simulink model "PKM_Planar_Testbench_2018"  (R2024a)
settings: Solver=FixedStepDiscrete  StartTime=0.0  StopTime=inf  FixedStep=param.t_sample  RelTol=1e-3
undefined symbols (not defined in the file or in its folder): max_qa, min_qa, param, slave3
libraries: Cust_Library_planarPKM x54, simulink_extras x27, dspswit3 x24, simulink x22, etherlab_lib x12
(part 4 of 6)

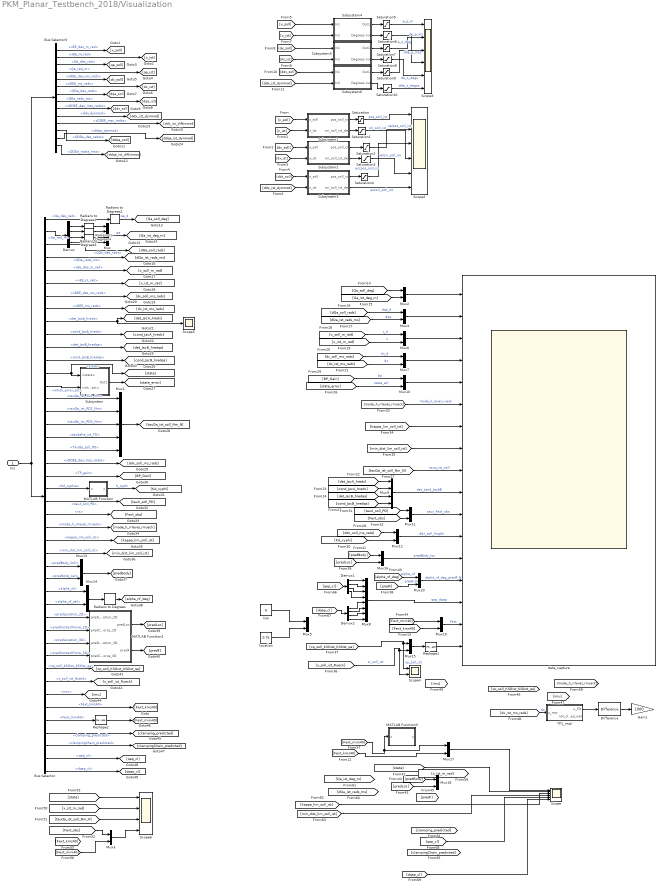
== system PKM_Planar_Testbench_2018/Visualization ==
  In1 : Inport
  Bus Selector : BusSelector  OutputSignals=Logical data.Qa_des_rad,Kinematics_currentValues.Qa_rad_m,Logical data.QDa_des_rads,Differential kinematics - current values.QDa_rads_ms,Logical data.xEE_des_m_rad,Kinematics_currentValues.xEE_m_rad,Logical data.xDEE_des_ms_rads,Differential kinematics - current values.xDEE_ms_rads,Differential kinematics - current values.det_JacA_hredx,Differential kinematics - current values.cond_JacA_hredx,Differential kinematics - current values.det_JacB_hredqa,Differential kinematics - current values.cond_JacB_hredqa,Logical data.state,Logical data.which_error_act,Messdaten.tauQa_ist_RD1_Nm,Messdaten.tauQa_ist_RD2_Nm,Messdaten.tauQa_ist_RD3_Nm,Messdaten.taudelta_ist_TD,PD_Controller.TauQa_soll_PD,Logical data.xDDEE_des_mss_radss,Controlpanel.TP_gain,PD_Controller.Kd_xyphie,PD_Controller.tauX_soll_PD,Beobachter.rx,PD_Controller.mode_h_rrlevel_rrrueck,PD_Controller.kappa_lim_soll_ist,PD_Controller.min_dist_lim_soll_ist,Beobachter.predBody_Coll,Beobachter.predbody_sel,Beobachter.alpha_nf,PD_Controller.alpha_nf_sel,Beobachter.predLocation_2D,Beobachter.predContactForce_2D,Beobachter.predLocation_3D,Beobachter.predContactForce_3D,PD_Controller.xp_soll_KSGist_KS0ist_qa,PD_Controller.x_soll_ist_Rueck,Messdaten.imu,Messdaten.Fext_kms40,Messdaten.Fext_mini40,Beobachter.clamping_predicted,Beobachter.clampingChain_predicted,PD_Controller.qap_cl,PD_Controller.dqap_cl
  Bus Selector3 : BusSelector  OutputSignals=Logical data.xEE_des_m_rad,Kinematics_currentValues.xEE_m_rad,Logical data.Qa_des_rad,Kinematics_currentValues.Qa_rad_m,Logical data.xDEE_des_ms_rads,Differential kinematics - current values.xDEE_ms_rads,Logical data.QDa_des_rads,Differential kinematics - current values.QDa_rads_ms,Logical data.xDDEE_des_mss_radss,Dynamik.ddx_dynmod,Differential kinematics - current values.xDDEE_mss_radss,Logical data.QDDa_des_radss,Dynamik.ddqa_dynmod,Differential kinematics - current values.QDDa_radss_mss
  Demux : Demux
  Demux1 : Demux
  Demux2 : Demux
  Difference : simulink/Discrete/Difference  ICPrevInput=0  OutMin=[]  OutMax=[]  OutDataType=fixdt(1, 16)  OutScaling=2^-10  DoSatur=off
  Gain1 : Gain  Gain=1000
  MATLAB Function : MATLAB Function  TreatAsAtomicUnit=on
  MATLAB Function2 : MATLAB Function  TreatAsAtomicUnit=on
  MATLAB Function3 : MATLAB Function  TreatAsAtomicUnit=on
  Mux : Mux
  Mux1 : Mux  Inputs=5
  Mux{2..7,10..20} (17 alike) : Mux  Inputs=2
  Mux8 : Mux  Inputs=8
  Mux9 : Mux
  Radians to Degrees{,1..4} (5 alike) : simulink_extras/Transformations/Radians to Degrees
  Reshape1 : Reshape
  Reshape2 : Reshape
  Saturation{,5,7,9} (4 alike) : Saturate  UpperLimit=0.35  LowerLimit=-0.35
  Saturation{1,3,6,8,10} (5 alike) : Saturate  UpperLimit=45  LowerLimit=-45
  Saturation2 : Saturate  UpperLimit=2  LowerLimit=-2
  Saturation4 : Saturate  UpperLimit=30  LowerLimit=-30
  Scope : Scope  NumInputPorts=6
  Scope2 : Scope  NumInputPorts=6
  Scope3 : Scope  NumInputPorts=6
  Scope4 : Scope  NumInputPorts=2
  Scope5 : Scope
  Scope6 : Scope  NumInputPorts=4
  Subsystem : Subsystem
  Subsystem1 : Subsystem
  Subsystem2 : Subsystem
  Subsystem3 : Subsystem
  Subsystem4 : Subsystem
  Subsystem5 : Subsystem
  Subsystem6 : Subsystem
  TP1_impl : Subsystem
  data_capture : Scope  NumInputPorts=17
  link : Constant  Value=6  SampleTime=-1
  location : Constant  Value=0.75  SampleTime=-1
  wires:
  Bus Selector/1 -> Radians to Degrees2/1  "<Qa_des_rad>"
  Bus Selector/16 -> Mux1/2  "<tauQa_ist_RD2_Nm>"
  Bus Selector/15 -> Mux1/1  "<tauQa_ist_RD1_Nm>"
  Bus Selector/17 -> Mux1/3  "<tauQa_ist_RD3_Nm>"
  Bus Selector/18 -> Mux1/4  "<taudelta_ist_TD>"
  Bus Selector/13 -> Subsystem/1(<state>), [state]  "<state>"
  Bus Selector/14 -> Subsystem/2(<which_error_act>)  "<which_error_act>"
  Bus Selector/22 -> MATLAB Function/1(u)  "<Kd_xyphie>"
  Bus Selector/24 -> [Fext_obs]  "<rx>"
  Bus Selector3/10 -> [ddx_ist_dynmod]  "<ddx_dynmod>"
  Bus Selector3/13 -> [ddqa_ist_dynmod]  "<ddqa_dynmod>"
  In1/1 -> Bus Selector3/1, Bus Selector/1
  Bus Selector3/1 -> [x_soll]  "<xEE_des_m_rad>"
  Bus Selector3/2 -> [x_ist]  "<xEE_m_rad>"
  Bus Selector3/3 -> [qa_soll]  "<Qa_des_rad>"
  Bus Selector3/4 -> [qa_ist]  "<Qa_rad_m>"
  Bus Selector3/6 -> [dx_ist]  "<xDEE_ms_rads>"
  Bus Selector3/5 -> [dx_soll]  "<xDEE_des_ms_rads>"
  Bus Selector3/7 -> [dqa_soll]  "<QDa_des_rads>"
  Bus Selector3/8 -> [dqa_ist]  "<QDa_rads_ms>"
  Bus Selector3/9 -> [ddx_soll]  "<xDDEE_des_mss_radss>"
  Bus Selector3/11 -> [ddx_ist_difkinmod]  "<xDDEE_mss_radss>"
  Bus Selector3/12 -> [ddqa_soll]  "<QDDa_des_radss>"
  Bus Selector3/14 -> [ddqa_ist_difkinmod]  "<QDDa_radss_mss>"
  [x_soll] -> Subsystem1/1(x_soll)
  [x_ist] -> Subsystem1/2(x_ist)
  [dx_ist] -> Subsystem2/2(x_ist)
  [dx_soll] -> Subsystem2/1(x_soll)
  [ddx_soll] -> Subsystem3/1(x_soll)
  [ddx_ist_dynmod] -> Subsystem3/2(x_ist)
  Subsystem1/1(pos_soll_ist) -> Saturation/1
  Subsystem2/1(pos_soll_ist) -> Saturation2/1
  Subsystem3/1(pos_soll_ist) -> Saturation4/1
  Subsystem1/2(ori_soll_ist_deg) -> Saturation1/1
  Subsystem2/2(ori_soll_ist_deg) -> Saturation3/1
  Subsystem3/2(ori_soll_ist_deg) -> Scope2/6  "accori_soll_ist"
  Saturation/1 -> Scope2/1  "pos_soll_ist"
  Saturation1/1 -> Scope2/4  "ori_soll_ist"
  Saturation2/1 -> Scope2/2  "velpos_soll_ist"
  Saturation3/1 -> Scope2/5  "velori_soll_ist"
  Saturation4/1 -> Scope2/3  "accpos_soll_ist"
  Saturation5/1 -> Scope3/1  "e_p_m"
  [x_soll] -> Subsystem4/1(In1)
  [x_ist] -> Subsystem4/2(In2)
  Subsystem4/1(Out1) -> Saturation5/1
  Subsystem4/2(Degrees out) -> Saturation6/1
  Saturation6/1 -> Scope3/4  "e_o_deg"
  Saturation8/1 -> Scope3/5  "de_o_degs"
  Subsystem5/2(Degrees out) -> Saturation8/1
  Subsystem5/1(Out1) -> Saturation7/1
  [dx_ist] -> Subsystem5/2(In2)
  [dx_soll] -> Subsystem5/1(In1)
  Saturation7/1 -> Scope3/2  "de_p_ms"
  Saturation9/1 -> Scope3/3  "dde_p_mss"
  [ddx_soll] -> Subsystem6/1(In1)
  [ddx_ist_dynmod] -> Subsystem6/2(In2)
  Subsystem6/1(Out1) -> Saturation9/1
  Subsystem6/2(Degrees out) -> Saturation10/1
  Saturation10/1 -> Scope3/6  "dde_o_degss"
  [Fext_mini40] -> MATLAB Function3/1(u), Mux17/1
  Radians to Degrees2/1 -> [Qa_soll_deg]  "qa_d"
  Bus Selector/3 -> [dQa_soll_rads]  "<QDa_des_rads>"
  Bus Selector/2 -> Demux/1  "<Qa_rad_m>"
  Demux/1 -> Radians to Degrees1/1
  Demux/2 -> Radians to Degrees3/1
  Demux/3 -> Radians to Degrees4/1
  Radians to Degrees4/1 -> Mux/3
  Radians to Degrees3/1 -> Mux/2
  Radians to Degrees1/1 -> Mux/1
  Demux/4 -> Mux/4
  Mux/1 -> [Qa_ist_deg_m]  "qa"
  Bus Selector/4 -> [dQa_ist_rads_ms]  "<QDa_rads_ms>"
  Bus Selector/5 -> [x_soll_m_rad]  "<xEE_des_m_rad>"
  Bus Selector/6 -> [x_ist_m_rad]  "<xEE_m_rad>"
  Bus Selector/7 -> [dx_soll_ms_rads]  "<xDEE_des_ms_rads>"
  Bus Selector/8 -> [dx_ist_ms_rads]  "<xDEE_ms_rads>"
  Bus Selector/9 -> Scope5/1, [det_JacA_hredx]  "<det_JacA_hredx>"
  Bus Selector/10 -> [cond_JacA_hredx]  "<cond_JacA_hredx>"
  Bus Selector/11 -> [det_JacB_hredqa]  "<det_JacB_hredqa>"
  Bus Selector/12 -> [cond_JacB_hredqa]  "<cond_JacB_hredqa>"
  Subsystem/1(Out1) -> [state_error]
  Mux1/1 -> [tauQa_ist_soll_Nm_N]
  Bus Selector/19 -> Mux1/5  "<TauQa_soll_PD>"
  Bus Selector/20 -> [ddx_soll_ms_rads]  "<xDDEE_des_mss_radss>"
  Bus Selector/21 -> [BP_Gain]  "<TP_gain>"
  MATLAB Function/1(y) -> [Kd_xyphi]  "K_xyphi"
  Bus Selector/23 -> [tauX_soll_PD]  "<tauX_soll_PD>"
  [Qa_soll_deg] -> Mux2/1
  [Qa_ist_deg_m] -> Mux2/2
  [dQa_soll_rads] -> Mux4/1  "dqa_d"
  [dQa_ist_rads_ms] -> Mux4/2  "dqa"
  [dx_ist_ms_rads] -> Mux7/2  "dx"
  [dx_soll_ms_rads] -> Mux7/1  "dx_d"
  [x_ist_m_rad] -> Mux6/2  "x"
  [x_soll_m_rad] -> Mux6/1  "x_d"
  [det_JacA_hredx] -> Mux9/1
  [cond_JacA_hredx] -> Mux9/2
  [det_JacB_hredqa] -> Mux9/3
  [cond_JacB_hredqa] -> Mux9/4
  Bus Selector/25 -> [mode_h_rrlevel_rrrueck]  "<mode_h_rrlevel_rrrueck>"
  Bus Selector/26 -> [kappa_lim_soll_ist]  "<kappa_lim_soll_ist>"
  Bus Selector/27 -> [min_dist_lim_soll_ist]  "<min_dist_lim_soll_ist>"
  Mux2/1 -> data_capture/1
  Mux4/1 -> data_capture/2
  Mux6/1 -> data_capture/3
  Mux7/1 -> data_capture/4
  [BP_Gain] -> Mux10/1  "bp"
  [state_error] -> Mux10/2  "state_err"
  [tauX_soll_PD] -> Mux11/1
  [Fext_obs] -> Mux11/2
  [ddx_soll_ms_rads] -> Mux12/1
  [Kd_xyphi] -> Mux12/2
  Mux10/1 -> data_capture/5
  [mode_h_rrlevel_rrrueck] -> data_capture/6  "mode_h_level_rueck"
  [kappa_lim_soll_ist] -> data_capture/7
  [min_dist_lim_soll_ist] -> data_capture/8
  [tauQa_ist_soll_Nm_N] -> data_capture/9  "tauq_ist_soll"
  Mux9/1 -> data_capture/10  "det_cond_JacAB"
  Mux11/1 -> data_capture/11  "taux_Fext_obs"
  Mux12/1 -> data_capture/12  "ddx_soll_Kxyphi"
  Bus Selector/28 -> Mux13/1  "<predBody_Coll>"
  Bus Selector/29 -> Mux13/2  "<predbody_sel>"
  Mux13/1 -> [predBody]
  Bus Selector/30 -> Mux14/1  "<alpha_nf>"
  Bus Selector/32 -> MATLAB Function2/1(predLocation_2D)  "<predLocation_2D>"
  Bus Selector/31 -> Mux14/2  "<alpha_nf_sel>"
  Mux14/1 -> Radians to Degrees/1
  Radians to Degrees/1 -> [alpha_nf_deg]
  Bus Selector/33 -> MATLAB Function2/2(predContactForce_2D)  "<predContactForce_2D>"
  Bus Selector/34 -> MATLAB Function2/3(predLocation_3D)  "<predLocation_3D>"
  Bus Selector/35 -> MATLAB Function2/4(predContactForce_3D)  "<predContactForce_3D>"
  MATLAB Function2/1(predLoc) -> [predLoc]
  MATLAB Function2/2(predF) -> [predF]
  Bus Selector/37 -> [x_soll_ist_Rueck]  "<x_soll_ist_Rueck>"
  [predBody] -> Mux16/1
  [predLoc] -> Mux16/2
  Mux16/1 -> data_capture/13  "predBody_loc"
  [Fext_kms40] -> Mux19/2
  Bus Selector/36 -> [xp_soll_KSGist_KS0ist_qa]  "<xp_soll_KSGist_KS0ist_qa>"
  [xp_soll_KSGist_KS0ist_qa] -> Scope4/1, Mux15/1  "xp_soll_ist"
  [x_soll_ist_Rueck] -> Scope4/2, Mux15/2  "xr_soll_ist"
  [state] -> Scope/2
  Mux17/1 -> Scope/1
  [predLoc] -> Mux18/2
  [predBody] -> Mux18/1
  Bus Selector/38 -> [imu]  "<imu>"
  [dx_ist_ms_rads] -> TP1_impl/1(u_raw)  "dx"
  TP1_impl/1(u_filt) -> Difference/1
  Difference/1 -> Gain1/1
  Mux15/1 -> Reshape1/1
  [x_ist_m_rad] -> Scope6/2
  [tauQa_ist_soll_Nm_N] -> Scope6/3
  [Fext_obs] -> Mux3/1
  [state] -> Scope6/1
  Mux19/1 -> data_capture/16  "Fext"
  [Fext_mini40] -> Mux19/1
  Bus Selector/39 -> [Fext_kms40]  "<Fext_kms40>"
  Bus Selector/40 -> Reshape2/1  "<Fext_mini40>"
  [Fext_mini40] -> Mux3/2
  Mux3/1 -> Scope6/4
  link/1 -> Mux5/1
  location/1 -> Mux5/2
  Reshape1/1 -> data_capture/17
  [kappa_lim_soll_ist] -> Scope/3
  [min_dist_lim_soll_ist] -> Scope/4
  Bus Selector/41 -> [clamping_predicted]  "<clamping_predicted>"
  Bus Selector/42 -> [clampingChain_predicted]  "<clampingChain_predicted>"
  [Fext_kms40] -> Mux17/2
  Bus Selector/43 -> [qap_cl]  "<qap_cl>"
  Bus Selector/44 -> [dqap_cl]  "<dqap_cl>"
  Reshape2/1 -> [Fext_mini40]
  [alpha_nf_deg] -> Mux20/1  "alpha_nf"
  [predF] -> Mux20/2  "predF_N"
  Mux20/1 -> data_capture/14  "alpha_nf_deg_predF_N"
  [qap_cl] -> Scope/5
  [dqap_cl] -> Scope/6
  [dqap_cl] -> Demux2/1
  Mux8/1 -> data_capture/15  "qap_dqap"
  [qap_cl] -> Demux1/1
  Demux1/1 -> Mux8/1
  Demux1/2 -> Mux8/2
  Demux1/3 -> Mux8/3
  Demux1/4 -> Mux8/4
  Demux2/1 -> Mux8/5
  Demux2/2 -> Mux8/6
  Demux2/3 -> Mux8/7
  Demux2/4 -> Mux8/8

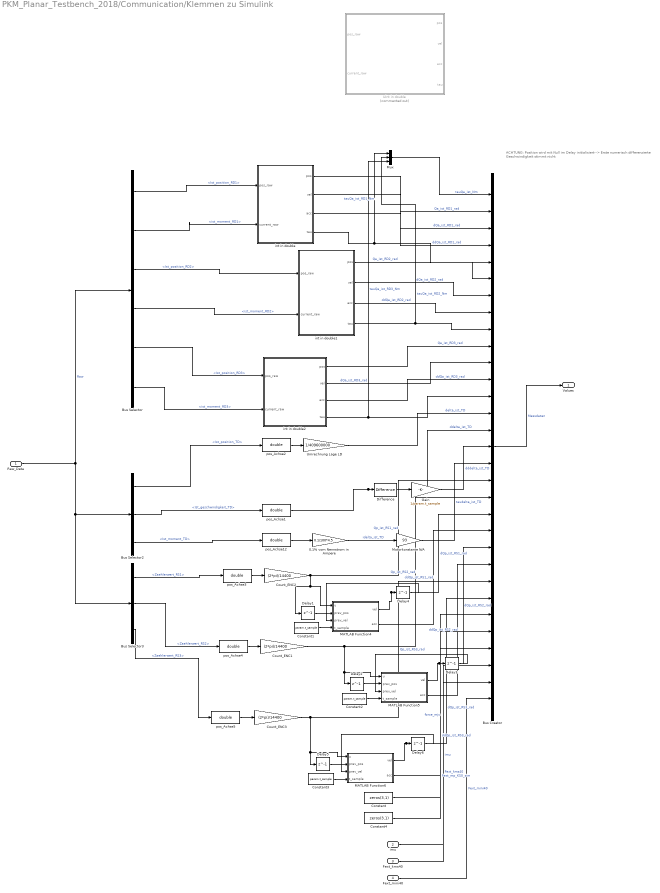
== system PKM_Planar_Testbench_2018/Communication/Klemmen zu Simulink ==
  note: ACHTUNG: Position wird mit Null im Delay initialisiert--> Erste numerisch differenzierte Geschwindigkeit stimmt nicht
  Raw_Data : Inport
  imu : Inport  Port=2
  Fext_kms40 : Inport  Port=3
  Fext_mini40 : Inport  Port=4
  0,1% vom Nennstrom in Ampere : Gain  Gain=0.1/100*4.5
  Bus Creator : BusCreator  Inputs=31
  Bus Selector : BusSelector  OutputSignals=Ist_position_RD1,ist_moment_RD1,Ist_position_RD2,ist_moment_RD2,Ist_position_RD3,ist_moment_RD3
  Bus Selector2 : BusSelector  OutputSignals=Ist_position_TD,Ist_geschwindigkeit_TD,Ist_moment_TD
  Bus Selector3 : BusSelector  OutputSignals=Zaehlerwert_RS1,Zaehlerwert_RS2,Zaehlerwert_RS3
  Constant : Constant  Value=zeros(3,1)  SampleTime=param.t_sample
  Constant1 : Constant  Value=param.t_sample  SampleTime=-1
  Constant2 : Constant  Value=param.t_sample  SampleTime=-1
  Constant3 : Constant  Value=param.t_sample  SampleTime=-1
  Constant4 : Constant  Value=zeros(3,1)  SampleTime=param.t_sample
  Count_ENC1 : Gain  Gain=(2*pi)/14400  ParamDataTypeStr=double  OutDataTypeStr=double
  Count_ENC2 : Gain  Gain=(2*pi)/14400  ParamDataTypeStr=double  OutDataTypeStr=double
  Count_ENC3 : Gain  Gain=(2*pi)/14400  ParamDataTypeStr=double  OutDataTypeStr=double
  Delay{1..6} (6 alike) : Delay  DelayLength=1
  Difference : simulink/Discrete/Difference  ICPrevInput=0.0  OutMin=[]  OutMax=[]  OutDataType=fixdt(1, 16)  OutScaling=2^-10  DoSatur=off
  Gain : Gain  Gain=1/param.t_sample
  MATLAB Function4 : MATLAB Function  TreatAsAtomicUnit=on
  MATLAB Function5 : MATLAB Function  TreatAsAtomicUnit=on
  MATLAB Function6 : MATLAB Function  TreatAsAtomicUnit=on
  Motorkonstante N/A : Gain  Gain=93
  Mux : Mux  Inputs=3
  Uint in double : Subsystem  Commented=on
  Umrechnung Lage LD : Gain  Gain=1/409600000
  int in double : Subsystem
  int in double1 : Subsystem
  int in double2 : Subsystem
  pos_Achse{1..5,12} (6 alike) : DataTypeConversion  OutDataTypeStr=double  SaturateOnIntegerOverflow=off  RndMeth=Floor
  Values : Outport
  wires:
  Raw_Data/1 -> Bus Selector3/1, Bus Selector2/1, Bus Selector/1  "Raw"
  Bus Creator/1 -> Values/1  "Messdaten"
  Bus Selector/1 -> int in double/1(pos_raw)  "<Ist_position_RD1>"
  Bus Selector/2 -> int in double/2(current_raw)  "<ist_moment_RD1>"
  int in double/1(pos) -> Bus Creator/2  "Qa_ist_RD1_rad"
  int in double/2(vel) -> Bus Creator/3  "dQa_ist_RD1_rad"
  int in double/3(acc) -> Bus Creator/4  "ddQa_ist_RD1_rad"
  int in double/4(tau) -> Bus Creator/5, Mux/1  "tauQa_ist_RD1_Nm"
  int in double1/4(tau) -> Bus Creator/9, Mux/2  "tauQa_ist_RD2_Nm"
  int in double1/3(acc) -> Bus Creator/8  "ddQa_ist_RD2_rad"
  int in double1/2(vel) -> Bus Creator/7  "dQa_ist_RD2_rad"
  int in double1/1(pos) -> Bus Creator/6  "Qa_ist_RD2_rad"
  Bus Selector/3 -> int in double1/1(pos_raw)  "<Ist_position_RD2>"
  Bus Selector/4 -> int in double1/2(current_raw)  "<ist_moment_RD2>"
  Bus Selector/5 -> int in double2/1(pos_raw)  "<Ist_position_RD3>"
  Bus Selector/6 -> int in double2/2(current_raw)  "<ist_moment_RD3>"
  int in double2/1(pos) -> Bus Creator/10  "Qa_ist_RD3_rad"
  int in double2/2(vel) -> Bus Creator/11  "dQa_ist_RD3_rad"
  int in double2/3(acc) -> Bus Creator/12  "ddQa_ist_RD3_rad"
  int in double2/4(tau) -> Mux/3, Bus Creator/13  "tauQa_ist_RD3_Nm"
  pos_Achse1/1 -> Difference/1, Bus Creator/15  "ddelta_ist_TD"
  Motorkonstante N/A/1 -> Bus Creator/17  "taudelta_ist_TD"
  pos_Achse2/1 -> Umrechnung Lage LD/1
  pos_Achse12/1 -> 0,1% vom Nennstrom in Ampere/1
  Bus Selector2/1 -> pos_Achse2/1  "<Ist_position_TD>"
  Bus Selector2/2 -> pos_Achse1/1  "<Ist_geschwindigkeit_TD>"
  Bus Selector2/3 -> pos_Achse12/1  "<Ist_moment_TD>"
  Umrechnung Lage LD/1 -> Bus Creator/14  "delta_ist_TD"
  pos_Achse3/1 -> Count_ENC2/1
  Count_ENC2/1 -> MATLAB Function4/1(u), Delay1/1, Bus Creator/18  "Qp_ist_RS1_rad"
  Bus Selector3/1 -> pos_Achse3/1  "<Zaehlerwert_RS1>"
  pos_Achse4/1 -> Count_ENC1/1
  pos_Achse5/1 -> Count_ENC3/1
  Count_ENC3/1 -> Delay5/1, MATLAB Function6/1(u), Bus Creator/24  "Qp_ist_RS3_rad"
  Bus Selector3/3 -> pos_Achse5/1  "<Zaehlerwert_RS3>"
  Bus Selector3/2 -> pos_Achse4/1  "<Zaehlerwert_RS2>"
  Count_ENC1/1 -> Delay2/1, MATLAB Function5/1(u), Bus Creator/19  "Qp_ist_RS2_rad"
  0,1% vom Nennstrom in Ampere/1 -> Motorkonstante N/A/1  "idelta_ist_TD"
  Difference/1 -> Gain/1
  Gain/1 -> Bus Creator/16  "dddelta_ist_TD"
  Delay1/1 -> MATLAB Function4/2(prev_pos)
  Constant1/1 -> MATLAB Function4/4(t_sample)
  Delay4/1 -> MATLAB Function4/3(prev_vel)
  MATLAB Function4/1(vel) -> Delay4/1, Bus Creator/20  "dQp_ist_RS1_rad"
  MATLAB Function4/2(acc) -> Bus Creator/21  "ddQp_ist_RS1_rad"
  Constant2/1 -> MATLAB Function5/4(t_sample)
  MATLAB Function5/1(vel) -> Bus Creator/22, Delay3/1  "dQp_ist_RS2_rad"
  Delay3/1 -> MATLAB Function5/3(prev_vel)
  Delay2/1 -> MATLAB Function5/2(prev_pos)
  MATLAB Function5/2(acc) -> Bus Creator/23  "ddQp_ist_RS2_rad"
  Constant3/1 -> MATLAB Function6/4(t_sample)
  MATLAB Function6/1(vel) -> Delay6/1, Bus Creator/25  "dQp_ist_RS3_rad"
  Delay6/1 -> MATLAB Function6/3(prev_vel)
  Delay5/1 -> MATLAB Function6/2(prev_pos)
  MATLAB Function6/2(acc) -> Bus Creator/26  "ddQp_ist_RS3_rad"
  Mux/1 -> Bus Creator/1  "tauQa_ist_Nm"
  Constant/1 -> Bus Creator/27  "force_mjc"
  Constant4/1 -> Bus Creator/28  "Fext_mp_KS0_sim"
  imu/1 -> Bus Creator/29  "imu"
  Fext_kms40/1 -> Bus Creator/30  "Fext_kms40"
  Fext_mini40/1 -> Bus Creator/31  "Fext_mini40"

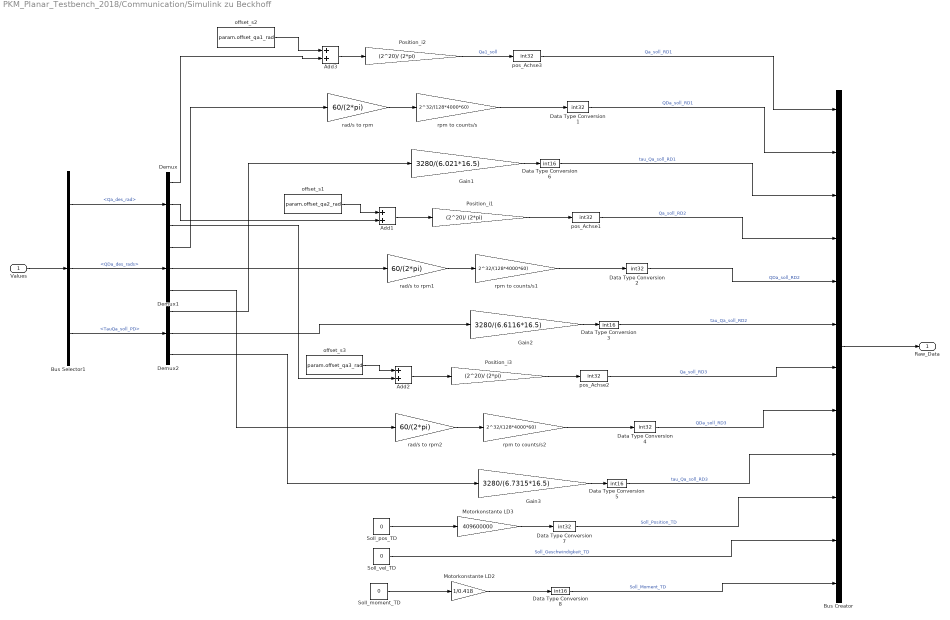
== system PKM_Planar_Testbench_2018/Communication/Simulink zu Beckhoff ==
  Values : Inport
  Add1 : Sum
  Add2 : Sum
  Add3 : Sum
  Bus Creator : BusCreator  Inputs=12
  Bus Selector1 : BusSelector  OutputSignals=Logical data.Qa_des_rad,Logical data.QDa_des_rads,PD_Controller.TauQa_soll_PD
  Data Type Conversion{1..2,4,7} (4 alike) : DataTypeConversion  OutDataTypeStr=int32  SaturateOnIntegerOverflow=off  RndMeth=Floor
  Data Type Conversion{3,5..6,8} (4 alike) : DataTypeConversion  OutDataTypeStr=int16  SaturateOnIntegerOverflow=off  RndMeth=Floor
  Demux : Demux  Outputs=3
  Demux1 : Demux  Outputs=3
  Demux2 : Demux  Outputs=3
  Gain1 : Gain  Gain=3280/(6.021*16.5)
  Gain2 : Gain  Gain=3280/(6.6116*16.5)
  Gain3 : Gain  Gain=3280/(6.7315*16.5)
  Motorkonstante LD2 : Gain  Gain=1/0.418
  Motorkonstante LD3 : Gain  Gain=409600000
  Position_i1 : Gain  Gain=(2^20)/ (2*pi)  ParamDataTypeStr=float('double')  OutDataTypeStr=float('double')
  Position_i2 : Gain  Gain=(2^20)/ (2*pi)  ParamDataTypeStr=float('double')  OutDataTypeStr=float('double')
  Position_i3 : Gain  Gain=(2^20)/ (2*pi)  ParamDataTypeStr=float('double')  OutDataTypeStr=float('double')
  Soll_moment_TD : Constant  Value=0  SampleTime=-1
  Soll_pos_TD : Constant  Value=0  SampleTime=-1
  Soll_vel_TD : Constant  Value=0  SampleTime=-1
  offset_s1 : Constant  Value=param.offset_qa2_rad  SampleTime=-1
  offset_s2 : Constant  Value=param.offset_qa1_rad  SampleTime=-1
  offset_s3 : Constant  Value=param.offset_qa3_rad  SampleTime=-1
  pos_Achse1 : DataTypeConversion  OutDataTypeStr=int32  SaturateOnIntegerOverflow=off  RndMeth=Floor
  pos_Achse2 : DataTypeConversion  OutDataTypeStr=int32  SaturateOnIntegerOverflow=off  RndMeth=Floor
  pos_Achse3 : DataTypeConversion  OutDataTypeStr=int32  SaturateOnIntegerOverflow=off  RndMeth=Floor
  rad/s to rpm : Gain  Gain=60/(2*pi)
  rad/s to rpm1 : Gain  Gain=60/(2*pi)
  rad/s to rpm2 : Gain  Gain=60/(2*pi)
  rpm to counts/s : Gain  Gain=2^32/(128*4000*60)
  rpm to counts/s1 : Gain  Gain=2^32/(128*4000*60)
  rpm to counts/s2 : Gain  Gain=2^32/(128*4000*60)
  Raw_Data : Outport
  wires:
  Demux1/1 -> rad/s to rpm/1
  Bus Creator/1 -> Raw_Data/1
  Gain1/1 -> Data Type Conversion6/1
  Demux2/1 -> Gain1/1
  Values/1 -> Bus Selector1/1
  Data Type Conversion1/1 -> Bus Creator/2  "QDa_soll_RD1"
  Data Type Conversion6/1 -> Bus Creator/3  "tau_Qa_soll_RD1"
  Demux/1 -> Add3/2
  Bus Selector1/1 -> Demux/1  "<Qa_des_rad>"
  Bus Selector1/2 -> Demux1/1  "<QDa_des_rads>"
  pos_Achse3/1 -> Bus Creator/1  "Qa_soll_RD1"
  rad/s to rpm/1 -> rpm to counts/s/1
  rpm to counts/s/1 -> Data Type Conversion1/1
  rpm to counts/s1/1 -> Data Type Conversion2/1
  rad/s to rpm1/1 -> rpm to counts/s1/1
  Gain2/1 -> Data Type Conversion3/1
  Demux/2 -> Add1/2
  Demux1/2 -> rad/s to rpm1/1
  Demux2/2 -> Gain2/1
  rad/s to rpm2/1 -> rpm to counts/s2/1
  Gain3/1 -> Data Type Conversion5/1
  rpm to counts/s2/1 -> Data Type Conversion4/1
  Demux/3 -> Add2/2
  Demux1/3 -> rad/s to rpm2/1
  Demux2/3 -> Gain3/1
  Data Type Conversion5/1 -> Bus Creator/9  "tau_Qa_soll_RD3"
  Data Type Conversion4/1 -> Bus Creator/8  "QDa_soll_RD3"
  pos_Achse2/1 -> Bus Creator/7  "Qa_soll_RD3"
  Data Type Conversion3/1 -> Bus Creator/6  "tau_Qa_soll_RD2"
  Data Type Conversion2/1 -> Bus Creator/5  "QDa_soll_RD2"
  pos_Achse1/1 -> Bus Creator/4  "Qa_soll_RD2"
  Soll_moment_TD/1 -> Motorkonstante LD2/1
  Soll_pos_TD/1 -> Motorkonstante LD3/1
  Motorkonstante LD3/1 -> Data Type Conversion7/1
  Motorkonstante LD2/1 -> Data Type Conversion8/1
  Data Type Conversion8/1 -> Bus Creator/12  "Soll_Moment_TD"
  Data Type Conversion7/1 -> Bus Creator/10  "Soll_Position_TD"
  Soll_vel_TD/1 -> Bus Creator/11  "Soll_Geschwindigkeit_TD"
  Position_i2/1 -> pos_Achse3/1  "Qa1_soll"
  Add3/1 -> Position_i2/1
  offset_s2/1 -> Add3/1
  Position_i1/1 -> pos_Achse1/1
  Add1/1 -> Position_i1/1
  offset_s1/1 -> Add1/1
  Position_i3/1 -> pos_Achse2/1
  Add2/1 -> Position_i3/1
  offset_s3/1 -> Add2/1
  Bus Selector1/3 -> Demux2/1  "<TauQa_soll_PD>"

== system PKM_Planar_Testbench_2018/Communication/voltage2force_torque ==
  In1 : Inport
  Add : Sum
  Demux : Demux  Outputs=6
  Display : Display
  Gewichtskraft : Constant  Value=param.Gewichtskraft  SampleTime=-1
  Product : Product  Multiplication=Matrix(*)  RndMeth=Zero
  Terminator1 : Terminator
  Vector Concatenate : Concatenate  NumInputs=6  Mode=Multidimensional array
  Vector Concatenate1 : Concatenate  NumInputs=6  Mode=Multidimensional array
  Working Matrix (Sensor Calibration ATI nano17 titanium) : Constant  Value=|  SampleTime=-1
      | [0.00224   0.02368   0.03529  -0.80632  -0.02445   0.81101;
      |     -0.03942   0.96116   0.01956  -0.43177   0.01604  -0.49865;
      | 	0.90808   0.00103   0.90339  -0.01514   0.94300   0.02877;
      | 	-0.45186   5.88481   5.15243  -2.71284  -5.03331  -3.21371;
      | 	-5.75693  -0.16648   2.68349   4.90294   3.39391  -4.86367;
      | 	-0.11787   3.34042  -0.17354   3.25781  -0.12176   3.65024;];
  Working Matrix (Sensor Calibration) : Constant  Value=|  SampleTime=-1
      | [0.052070987 -0.130514746 0.961791687 12.71279467 -0.63882202 -11.78736376;
      | -1.115563222 -14.4308958 0.66281852 7.178188359 0.390451919 7.011768932;
      | 21.03335044 1.08132865 20.50422466 -0.287397369 21.07979804 -1.27937419;
      | -0.012415733 -0.080850353 0.29706849 0.038847671 -0.303166527 0.053776337;
      | -0.337109545 -0.019553002 0.16260793 -0.070950006 0.180720365 0.05582245;
      | -0.010311409 -0.169646682 -0.011904742 -0.173975353 -0.011770042 -0.165476508]
  Zero-Order Hold : ZeroOrderHold  SampleTime=-1
  Zero-Order Hold1 : ZeroOrderHold  SampleTime=-1
  biasFT : Constant  SampleTime=-1
  mittelwert1 : MATLAB Function  TreatAsAtomicUnit=on
  mittelwert2 : MATLAB Function  TreatAsAtomicUnit=on
  mittelwert3 : MATLAB Function  TreatAsAtomicUnit=on
  mittelwert4 : MATLAB Function  TreatAsAtomicUnit=on
  mittelwert5 : MATLAB Function  TreatAsAtomicUnit=on
  mittelwet2 : MATLAB Function  TreatAsAtomicUnit=on
  FT : Outport  VectorParamsAs1DForOutWhenUnconnected=off
  V_unbiased : Outport  Port=2  VectorParamsAs1DForOutWhenUnconnected=off
  wires:
  Demux/2 -> mittelwert4/1(u)
  mittelwert2/2(mittelwert) -> Vector Concatenate1/4
  Demux/3 -> mittelwert3/1(u)
  Demux/5 -> mittelwet2/1(u)
  mittelwert1/1(y) -> Vector Concatenate/6
  mittelwert3/2(mittelwert) -> Vector Concatenate1/3
  mittelwert2/1(y) -> Vector Concatenate/4
  mittelwert5/2(mittelwert) -> Vector Concatenate1/1
  mittelwert5/1(y) -> Vector Concatenate/1
  mittelwert3/1(y) -> Vector Concatenate/3
  mittelwert4/1(y) -> Vector Concatenate/2
  Demux/6 -> mittelwert1/1(u)
  Demux/4 -> mittelwert2/1(u)
  mittelwet2/1(y) -> Vector Concatenate/5
  Demux/1 -> mittelwert5/1(u)
  In1/1 -> Demux/1
  mittelwert1/2(mittelwert) -> Vector Concatenate1/6
  mittelwert4/2(mittelwert) -> Vector Concatenate1/2
  mittelwet2/2(mittelwert) -> Vector Concatenate1/5
  Zero-Order Hold/1 -> mittelwert1/2(set_zero), mittelwet2/2(set_zero), mittelwert2/2(set_zero), mittelwert3/2(set_zero), mittelwert4/2(set_zero), mittelwert5/2(set_zero)
  Zero-Order Hold1/1 -> Product/1
  Vector Concatenate/1 -> V_unbiased/1, Product/2
  Vector Concatenate1/1 -> Display/1
  Product/1 -> Add/1
  Add/1 -> FT/1
  biasFT/1 -> Zero-Order Hold/1
  Gewichtskraft/1 -> Add/2
  Working Matrix (Sensor Calibration)/1 -> Zero-Order Hold1/1
  Working Matrix (Sensor Calibration ATI nano17 titanium)/1 -> Terminator1/1

== system PKM_Planar_Testbench_2018/Control/TP1_impl ==
  u_raw : Inport
  Constant16 : Constant  Value=param.fz_lp  SampleTime=-1
  Delay5 : Delay  DelayLength=1  InitialCondition=zeros(3,1)
  Delay6 : Delay  DelayLength=1  InitialCondition=zeros(3,1)
  MATLAB Function16 : MATLAB Function  TreatAsAtomicUnit=on
  "TP1_scope " : Scope  NumInputPorts=5
  u_filt : Outport
  not_defined_nan : Outport  Port=2
  wires:
  Delay5/1 -> "TP1_scope "/2, MATLAB Function16/2(u_prev)
  u_raw/1 -> Delay5/1, "TP1_scope "/1, MATLAB Function16/1(u_raw)
  MATLAB Function16/1(u_filt) -> "TP1_scope "/4, u_filt/1, Delay6/1
  Constant16/1 -> "TP1_scope "/3, MATLAB Function16/3(a)
  Delay6/1 -> "TP1_scope "/5, MATLAB Function16/4(y_prev)
  MATLAB Function16/2(not_defined_nan) -> not_defined_nan/1

== system PKM_Planar_Testbench_2018/Control/TP1_impl10 ==
  u_raw : Inport
  Constant16 : Constant  Value=2/ (2*pi*param.f_lp_Hz*param.t_sample)  SampleTime=-1
  Delay5 : Delay  DelayLength=1  InitialCondition=zeros(1,3)
  Delay6 : Delay  DelayLength=1  InitialCondition=zeros(1,3)
  MATLAB Function16 : MATLAB Function  TreatAsAtomicUnit=on
  "TP1_scope " : Scope  NumInputPorts=6
  u_filt : Outport
  wires:
  Delay5/1 -> "TP1_scope "/2, MATLAB Function16/2(u_prev_)
  u_raw/1 -> Delay5/1, "TP1_scope "/1, MATLAB Function16/1(u_raw)
  MATLAB Function16/1(u_filt) -> "TP1_scope "/4, u_filt/1, Delay6/1
  Constant16/1 -> "TP1_scope "/3, MATLAB Function16/3(a)
  Delay6/1 -> "TP1_scope "/5, MATLAB Function16/4(y_prev_)
  MATLAB Function16/2(not_defined_nan) -> "TP1_scope "/6

== system PKM_Planar_Testbench_2018/Control/TP1_impl9 ==
  u_raw : Inport
  Constant16 : Constant  Value=2/ (2*pi*param.f_lp_Hz*param.t_sample)  SampleTime=-1
  Delay5 : Delay  DelayLength=1  InitialCondition=zeros(1,3)
  Delay6 : Delay  DelayLength=1  InitialCondition=zeros(1,3)
  MATLAB Function16 : MATLAB Function  TreatAsAtomicUnit=on
  "TP1_scope " : Scope  NumInputPorts=6
  u_filt : Outport
  wires:
  MATLAB Function16/2(not_defined_nan) -> "TP1_scope "/6
  Delay6/1 -> MATLAB Function16/4(y_prev_), "TP1_scope "/5
  Constant16/1 -> MATLAB Function16/3(a), "TP1_scope "/3
  MATLAB Function16/1(u_filt) -> Delay6/1, u_filt/1, "TP1_scope "/4
  u_raw/1 -> MATLAB Function16/1(u_raw), "TP1_scope "/1, Delay5/1
  Delay5/1 -> MATLAB Function16/2(u_prev_), "TP1_scope "/2

== system PKM_Planar_Testbench_2018/Control/Triggered Subsystem ==
  In1 : Inport
  Trigger : TriggerPort  VariantControl=Variant
  reaction_angle_rad : Outport
  wires:
  In1/1 -> reaction_angle_rad/1

== system PKM_Planar_Testbench_2018/Logic/Hold Configuration after enabling1 ==
  Theta_ist : Inport
  Trigger : TriggerPort  TriggerType=either  VariantControl=Variant
  "vec_x_0_Startposition " : Outport
  wires:
  Theta_ist/1 -> "vec_x_0_Startposition "/1

== system PKM_Planar_Testbench_2018/Logic/Hold Configuration after enabling2 ==
  x_ist_retr : Inport
  Trigger : TriggerPort  VariantControl=Variant
  "x_ist_retr_trigg " : Outport
  wires:
  x_ist_retr/1 -> "x_ist_retr_trigg "/1

== system PKM_Planar_Testbench_2018/Logic/Hold Configuration after enabling3 ==
  Theta_ist : Inport
  Trigger : TriggerPort  TriggerType=either  VariantControl=Variant
  "vec_x_0_Startposition " : Outport
  wires:
  Theta_ist/1 -> "vec_x_0_Startposition "/1

== system PKM_Planar_Testbench_2018/Logic/Hold Configuration after enabling4 ==
  x_ist_retr : Inport
  Trigger : TriggerPort  VariantControl=Variant
  "x_ist_retr_trigg " : Outport
  wires:
  x_ist_retr/1 -> "x_ist_retr_trigg "/1

== system PKM_Planar_Testbench_2018/Logic/Hold Configuration after enabling5 ==
  Theta_ist : Inport
  Trigger : TriggerPort  VariantControl=Variant
  "vec_x_0_Startposition " : Outport
  wires:
  Theta_ist/1 -> "vec_x_0_Startposition "/1

== system PKM_Planar_Testbench_2018/Logic/Hold Configuration after enabling6 ==
  Theta_ist : Inport
  Trigger : TriggerPort  VariantControl=Variant
  "vec_x_0_Startposition " : Outport
  wires:
  Theta_ist/1 -> "vec_x_0_Startposition "/1

== system PKM_Planar_Testbench_2018/Logic/Hold Configuration after enabling7 ==
  Theta_ist : Inport
  Trigger : TriggerPort  VariantControl=Variant
  "vec_x_0_Startposition " : Outport
  wires:
  Theta_ist/1 -> "vec_x_0_Startposition "/1

== system PKM_Planar_Testbench_2018/Logic/Hold Configuration after enabling8 ==
  qap_retr : Inport
  Trigger : TriggerPort  VariantControl=Variant
  "qap_retr_trig " : Outport
  wires:
  qap_retr/1 -> "qap_retr_trig "/1

== system PKM_Planar_Testbench_2018/Logic/Hold Configuration after enabling9 ==
  Theta_ist : Inport
  Trigger : TriggerPort  VariantControl=Variant
  "vec_x_0_Startposition " : Outport
  wires:
  Theta_ist/1 -> "vec_x_0_Startposition "/1

== system PKM_Planar_Testbench_2018/Logic/Hold initial position as target value for PD_Controller  ==
  Theta_ist : Inport
  Trigger : TriggerPort  TriggerType=either  VariantControl=Variant
  "vec_x_0_Startposition " : Outport
  wires:
  Theta_ist/1 -> "vec_x_0_Startposition "/1

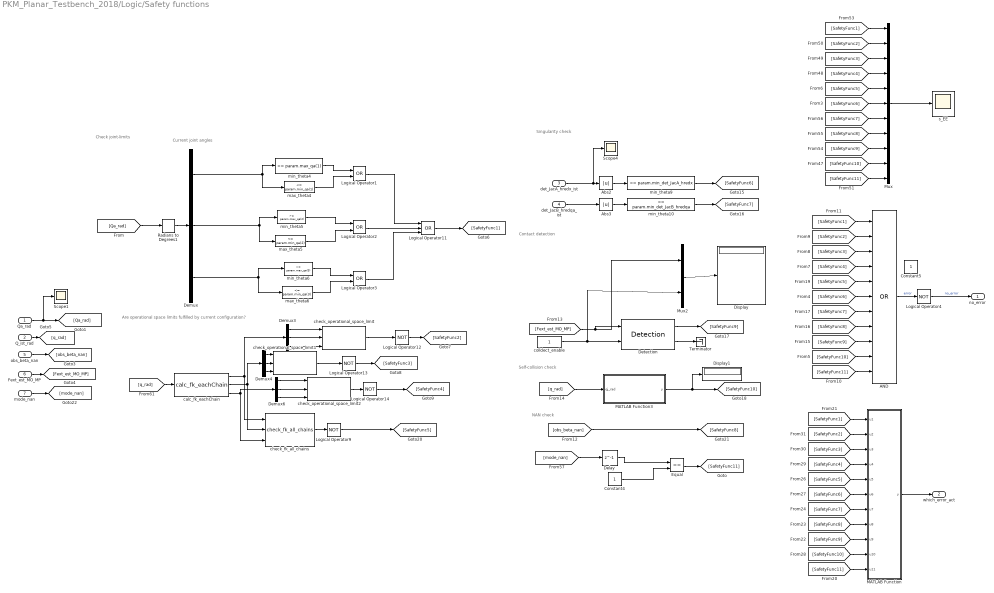
== system PKM_Planar_Testbench_2018/Logic/Safety functions ==
  note: Self-collision check
  note: Contact detection
  note: NAN check
  note: Singularity check
  note: Are operational space limits fulfilled by current configuration?
  note: Check joint-limits
  note: Current joint angles
  Qa_rad : Inport
  Q_ist_rad : Inport  Port=2
  det_JacA_hredx_ist : Inport  Port=3
  det_JacB_hredqa_ist : Inport  Port=4
  obs_beta_nan : Inport  Port=5
  Fext_est_MO_MP : Inport  Port=6
  mode_nan : Inport  Port=7
  AND : Logic  Operator=OR  Inputs=11  AllPortsSameDT=off  OutDataTypeStr=boolean
  Abs2 : Abs  SaturateOnIntegerOverflow=off
  Abs3 : Abs  SaturateOnIntegerOverflow=off
  Constant4 : Constant  SampleTime=-1
  Constant5 : Constant  SampleTime=-1
  Delay : Delay  DelayLength=1
  Demux{,3..4,6} (4 alike) : Demux  Outputs=3
  Detection : Cust_Library_planarPKM/Detection  ColDet_thresholds=param.CollDet_limit_MobPlat
  Display : Display
  Display1 : Display
  Equal : RelationalOperator  Operator===  OutDataTypeStr=boolean  RndMeth=Simplest  InputSameDT=off
  Logical Operator1 : Logic  Operator=OR  AllPortsSameDT=off  OutDataTypeStr=boolean
  Logical Operator11 : Logic  Operator=OR  Inputs=3  AllPortsSameDT=off  OutDataTypeStr=boolean
  Logical Operator{4,9,12..14} (5 alike) : Logic  Operator=NOT  Inputs=3  AllPortsSameDT=off  OutDataTypeStr=boolean
  Logical Operator2 : Logic  Operator=OR  AllPortsSameDT=off  OutDataTypeStr=boolean
  Logical Operator3 : Logic  Operator=OR  AllPortsSameDT=off  OutDataTypeStr=boolean
  MATLAB Function : MATLAB Function  TreatAsAtomicUnit=on
  MATLAB Function3 : MATLAB Function  TreatAsAtomicUnit=on
  Mux : Mux  Inputs=11
  Mux2 : Mux  Inputs=2
  Radians to Degrees1 : simulink_extras/Transformations/Radians to Degrees
  Scope1 : Scope
  Scope4 : Scope
  Terminator : Terminator
  calc_fk_eachChain : Cust_Library_planarPKM/calc_fk_eachChain  psi_j=param.psi_j  beta_j=param.beta_j  r_fixPlat_j=param.r_fixPlat_j  r_mobPlat_j=param.r_mobPlat_j  l_all_id=param.l_all_id
  check_fk_all_chains : Cust_Library_planarPKM/check_fk_all_chains  maxerrx=param.maxerrx  maxerry=param.maxerry
  check_operational_space_limit : Cust_Library_planarPKM/check_operational_space_limit  max_radius=param.max_radius  max_phie=param.max_phie
  check_operational_space_limit1 : Cust_Library_planarPKM/check_operational_space_limit  max_radius=param.max_radius  max_phie=param.max_phie
  check_operational_space_limit2 : Cust_Library_planarPKM/check_operational_space_limit  max_radius=param.max_radius  max_phie=param.max_phie
  colldect_enable : Constant  SampleTime=-1
  max_theta4 : simulink/Logic and Bit Operations/Compare To Constant  relop=<=  const=param.min_qa(1)  OutDataTypeStr=boolean
  max_theta5 : simulink/Logic and Bit Operations/Compare To Constant  relop=<=  const=param.min_qa(2)  OutDataTypeStr=boolean
  max_theta6 : simulink/Logic and Bit Operations/Compare To Constant  relop=<=  const=param.min_qa(3)  OutDataTypeStr=boolean
  min_theta10 : simulink/Logic and Bit Operations/Compare To Constant  relop=<=  const=param.min_det_JacB_hredqa  OutDataTypeStr=boolean
  min_theta4 : simulink/Logic and Bit Operations/Compare To Constant  relop=>=  const=param.max_qa(1)  OutDataTypeStr=boolean
  min_theta5 : simulink/Logic and Bit Operations/Compare To Constant  relop=>=  const=param.max_qa(2)  OutDataTypeStr=boolean
  min_theta6 : simulink/Logic and Bit Operations/Compare To Constant  relop=>=  const=param.max_qa(3)  OutDataTypeStr=boolean
  min_theta9 : simulink/Logic and Bit Operations/Compare To Constant  relop=<=  const=param.min_det_JacA_hredx  OutDataTypeStr=boolean
  s_EE : Scope
  no_error : Outport  VectorParamsAs1DForOutWhenUnconnected=off
  which_error_act : Outport  Port=2  VectorParamsAs1DForOutWhenUnconnected=off
  wires:
  AND/1 -> Logical Operator4/1  "error"
  Qa_rad/1 -> [Qa_rad], Scope1/1
  Logical Operator4/1 -> no_error/1  "no_error"
  Logical Operator11/1 -> [SafetyFunc1]
  Radians to Degrees1/1 -> Demux/1
  Logical Operator2/1 -> Logical Operator11/2
  Logical Operator3/1 -> Logical Operator11/3
  max_theta5/1 -> Logical Operator2/2
  max_theta6/1 -> Logical Operator3/2
  min_theta6/1 -> Logical Operator3/1
  Demux/2 -> min_theta5/1, max_theta5/1
  min_theta4/1 -> Logical Operator1/1
  Demux/3 -> max_theta6/1, min_theta6/1
  min_theta5/1 -> Logical Operator2/1
  Logical Operator1/1 -> Logical Operator11/1
  Demux/1 -> max_theta4/1, min_theta4/1
  max_theta4/1 -> Logical Operator1/2
  Q_ist_rad/1 -> [q_rad]
  Demux3/1 -> check_operational_space_limit/1
  Demux3/3 -> check_operational_space_limit/3
  Demux3/2 -> check_operational_space_limit/2
  calc_fk_eachChain/1 -> Demux3/1, check_fk_all_chains/1
  Demux4/2 -> check_operational_space_limit1/2
  Demux4/3 -> check_operational_space_limit1/3
  calc_fk_eachChain/2 -> Demux4/1, check_fk_all_chains/2
  Demux4/1 -> check_operational_space_limit1/1
  Demux6/2 -> check_operational_space_limit2/2
  Demux6/3 -> check_operational_space_limit2/3
  calc_fk_eachChain/3 -> Demux6/1, check_fk_all_chains/3
  Demux6/1 -> check_operational_space_limit2/1
  check_operational_space_limit/1 -> Logical Operator12/1
  check_operational_space_limit2/1 -> Logical Operator14/1
  check_operational_space_limit1/1 -> Logical Operator13/1
  Logical Operator12/1 -> [SafetyFunc2]
  Logical Operator13/1 -> [SafetyFunc3]
  Logical Operator14/1 -> [SafetyFunc4]
  det_JacA_hredx_ist/1 -> Scope4/1, Abs2/1
  det_JacB_hredqa_ist/1 -> Abs3/1
  Abs2/1 -> min_theta9/1
  Abs3/1 -> min_theta10/1
  min_theta9/1 -> [SafetyFunc6]
  min_theta10/1 -> [SafetyFunc7]
  check_fk_all_chains/1 -> Logical Operator9/1
  Logical Operator9/1 -> [SafetyFunc5]
  MATLAB Function/1(y) -> which_error_act/1
  obs_beta_nan/1 -> [obs_beta_nan]
  Fext_est_MO_MP/1 -> [Fext_est_MO_MP]
  [Fext_est_MO_MP] -> Mux2/1, Detection/1
  colldect_enable/1 -> Mux2/2, Detection/2
  Mux2/1 -> Display/1
  [q_rad] -> MATLAB Function3/1(qj_rad)
  MATLAB Function3/1(y) -> Display1/1, [SafetyFunc10]
  [Qa_rad] -> Radians to Degrees1/1
  [obs_beta_nan] -> [SafetyFunc8]
  Mux/1 -> s_EE/1
  Detection/1 -> [SafetyFunc9]
  mode_nan/1 -> [mode_nan]
  [mode_nan] -> Delay/1
  Constant4/1 -> Equal/2
  Equal/1 -> [SafetyFunc11]
  Delay/1 -> Equal/1
  [q_rad] -> calc_fk_eachChain/1
  Detection/2 -> Terminator/1
  [SafetyFunc1] -> Mux/1
  [SafetyFunc2] -> Mux/2
  [SafetyFunc3] -> Mux/3
  [SafetyFunc4] -> Mux/4
  [SafetyFunc5] -> Mux/5
  [SafetyFunc6] -> Mux/6
  [SafetyFunc7] -> Mux/7
  [SafetyFunc8] -> Mux/8
  [SafetyFunc9] -> Mux/9
  [SafetyFunc10] -> Mux/10
  [SafetyFunc11] -> Mux/11
  [SafetyFunc11] -> AND/11
  [SafetyFunc10] -> AND/10
  [SafetyFunc9] -> AND/9
  [SafetyFunc8] -> AND/8
  [SafetyFunc7] -> AND/7
  [SafetyFunc6] -> AND/6
  [SafetyFunc5] -> AND/5
  [SafetyFunc4] -> AND/4
  [SafetyFunc3] -> AND/3
  [SafetyFunc2] -> AND/2
  [SafetyFunc1] -> AND/1
  [SafetyFunc1] -> MATLAB Function/1(u1)
  [SafetyFunc2] -> MATLAB Function/2(u2)
  [SafetyFunc3] -> MATLAB Function/3(u3)
  [SafetyFunc4] -> MATLAB Function/4(u4)
  [SafetyFunc5] -> MATLAB Function/5(u5)
  [SafetyFunc6] -> MATLAB Function/6(u6)
  [SafetyFunc7] -> MATLAB Function/7(u7)
  [SafetyFunc8] -> MATLAB Function/8(u8)
  [SafetyFunc9] -> MATLAB Function/9(u9)
  [SafetyFunc10] -> MATLAB Function/10(u10)
  [SafetyFunc11] -> MATLAB Function/11(u11)

== system PKM_Planar_Testbench_2018/Logic/Trajectory ==
  tr_run : Inport
  Acceleration : Subsystem
  Counter1 : dspswit3/Counter  Direction=Up  CountEvent=Free running  CounterSize=32 bits  MaxCount=255  InitialCount=1  Output=Count  HitValue=32  ResetInput=on  SamplesPerFrame=1  Ts=-1  CntDtype=uint32  HitDtype=Logical
  Edge Detector1 : dspswit3/Edge Detector  InputProcessing=Columns as channels (frame based)
  Pose : Subsystem
  Trajectory_Length : Constant  Value=2302  SampleTime=-1
  Velocity : Subsystem
  pos_soll : Outport
  vel_soll : Outport  Port=2
  acc_soll : Outport  Port=3
  tr_isCalculating : Outport  Port=4
  XE0_soll : Outport  Port=5
  tr_valid : Outport  Port=6
  wires:
  Acceleration/1(XDDE_soll) -> acc_soll/1
  Pose/2(tr_isCalculating) -> tr_isCalculating/1
  Pose/3(XE0_soll) -> XE0_soll/1
  tr_run/1 -> Edge Detector1/1, Acceleration/1(tr_run), Velocity/1(tr_run), Pose/1(tr_run)
  Trajectory_Length/1 -> Acceleration/3(traj_length), Velocity/3(traj_length), Pose/3(traj_length)
  Edge Detector1/1 -> Counter1/1
  Counter1/1 -> Acceleration/2(Counter), Velocity/2(Counter), Pose/2(Counter)
  Velocity/1(XDE_soll) -> vel_soll/1
  Pose/1(XE_soll) -> pos_soll/1
  Pose/4(tr_valid) -> tr_valid/1

== system PKM_Planar_Testbench_2018/Logic/Validation of the EE end target pose ==
  XE_soll_relab : Inport
  Q_ist_rad : Inport  Port=2
  xEE_ist_m_rad : Inport  Port=3
  AND1 : Logic  Inputs=3  AllPortsSameDT=off  OutDataTypeStr=boolean
  Demux : Demux  Outputs=3
  MATLAB Function11 : MATLAB Function  TreatAsAtomicUnit=on
  Scope : Scope  NumInputPorts=3
  kinematic_invers : MATLAB Function  TreatAsAtomicUnit=on
  komplettes Q über rot ZBen aufstellen : MATLAB Function  TreatAsAtomicUnit=on
  taskspace_limitation : MATLAB Function  TreatAsAtomicUnit=on
  valid_invers_kinematic1 : Subsystem
  XE_end : Outport  VectorParamsAs1DForOutWhenUnconnected=off
  BP_valid : Outport  Port=2
  wires:
  Demux/3 -> taskspace_limitation/3(phie)
  Demux/2 -> taskspace_limitation/2(ye)
  Demux/1 -> taskspace_limitation/1(xe)
  kinematic_invers/1(qa) -> valid_invers_kinematic1/1(theta_in), komplettes Q über rot ZBen aufstellen/1(qa)
  XE_soll_relab/1 -> [xEE_soll], XE_end/1, Demux/1, kinematic_invers/1(xEE)
  valid_invers_kinematic1/1(kinematic_valid) -> Scope/2, AND1/2
  taskspace_limitation/1(euclid_valid) -> Scope/1, AND1/1
  AND1/1 -> BP_valid/1
  kinematic_invers/2(qp) -> komplettes Q über rot ZBen aufstellen/2(qp)
  Q_ist_rad/1 -> MATLAB Function11/1(qj_rad)
  xEE_ist_m_rad/1 -> MATLAB Function11/2(xEE_)
  [xEE_soll] -> komplettes Q über rot ZBen aufstellen/3(xEE)
  komplettes Q über rot ZBen aufstellen/1(q) -> [qj_rad_soll]
  [qj_rad_soll] -> MATLAB Function11/3(qj_soll)
  [xEE_soll] -> MATLAB Function11/4(xEE_soll_)
  MATLAB Function11/1(y) -> AND1/3, Scope/3  "det_JacA_hredx"

== system PKM_Planar_Testbench_2018/Observer/Triggered Subsystem ==
  In1 : Inport
  In2 : Inport  Port=2
  In3 : Inport  Port=3
  In4 : Inport  Port=4
  In5 : Inport  Port=5
  In6 : Inport  Port=6
  In7 : Inport  Port=7
  Trigger : TriggerPort  VariantControl=Variant
  out : Outport
  out1 : Outport  Port=2
  out2 : Outport  Port=3
  out3 : Outport  Port=4
  out4 : Outport  Port=5
  out5 : Outport  Port=6
  out6 : Outport  Port=7
  wires:
  In1/1 -> out/1
  In2/1 -> out1/1
  In3/1 -> out2/1
  In4/1 -> out3/1
  In5/1 -> out4/1
  In6/1 -> out5/1
  In7/1 -> out6/1

== system PKM_Planar_Testbench_2018/Observer/Triggered Subsystem1 ==
  In1 : Inport
  In2 : Inport  Port=2
  In3 : Inport  Port=3
  In4 : Inport  Port=4
  In5 : Inport  Port=5
  In6 : Inport  Port=6
  Trigger : TriggerPort  VariantControl=Variant
  out : Outport
  out1 : Outport  Port=2
  out2 : Outport  Port=3
  out3 : Outport  Port=4
  out4 : Outport  Port=5
  out5 : Outport  Port=6
  wires:
  In1/1 -> out/1
  In2/1 -> out1/1
  In4/1 -> out3/1
  In3/1 -> out2/1
  In5/1 -> out4/1
  In6/1 -> out5/1

== system PKM_Planar_Testbench_2018/Visualization/Subsystem ==
  <state> : Inport
  <which_error_act> : Inport  Port=2
  Demux2 : Demux  Outputs=11
  Mux4 : Mux  Inputs=12
  Out1 : Outport
  wires:
  Demux2/9 -> Mux4/10
  Demux2/7 -> Mux4/8
  Demux2/5 -> Mux4/6
  Demux2/1 -> Mux4/2
  Demux2/4 -> Mux4/5
  Demux2/11 -> Mux4/12
  Demux2/10 -> Mux4/11
  Demux2/6 -> Mux4/7
  Demux2/8 -> Mux4/9
  Demux2/2 -> Mux4/3
  Demux2/3 -> Mux4/4
  <which_error_act>/1 -> Demux2/1
  Mux4/1 -> Out1/1
  <state>/1 -> Mux4/1

== system PKM_Planar_Testbench_2018/Visualization/Subsystem1 ==
  x_soll : Inport
  x_ist : Inport  Port=2
  Demux : Demux  Outputs=3
  Demux1 : Demux  Outputs=3
  Mux10 : Mux  Inputs=2
  Mux9 : Mux
  Radians to Degrees : simulink_extras/Transformations/Radians to Degrees
  Radians to Degrees3 : simulink_extras/Transformations/Radians to Degrees
  pos_soll_ist : Outport
  ori_soll_ist_deg : Outport  Port=2
  wires:
  Demux/3 -> Radians to Degrees/1
  x_ist/1 -> Demux1/1
  Demux1/1 -> Mux9/2
  Radians to Degrees3/1 -> Mux10/2
  Demux1/2 -> Mux9/4
  Demux1/3 -> Radians to Degrees3/1
  Demux/1 -> Mux9/1
  Demux/2 -> Mux9/3
  Radians to Degrees/1 -> Mux10/1
  x_soll/1 -> Demux/1
  Mux10/1 -> ori_soll_ist_deg/1
  Mux9/1 -> pos_soll_ist/1

== system PKM_Planar_Testbench_2018/Visualization/Subsystem2 ==
  x_soll : Inport
  x_ist : Inport  Port=2
  Demux : Demux  Outputs=3
  Demux1 : Demux  Outputs=3
  Mux10 : Mux  Inputs=2
  Mux9 : Mux
  Radians to Degrees : simulink_extras/Transformations/Radians to Degrees
  Radians to Degrees3 : simulink_extras/Transformations/Radians to Degrees
  pos_soll_ist : Outport
  ori_soll_ist_deg : Outport  Port=2
  wires:
  Mux9/1 -> pos_soll_ist/1
  Mux10/1 -> ori_soll_ist_deg/1
  x_soll/1 -> Demux/1
  Radians to Degrees/1 -> Mux10/1
  Demux/2 -> Mux9/3
  Demux/1 -> Mux9/1
  Demux1/3 -> Radians to Degrees3/1
  Demux1/2 -> Mux9/4
  Radians to Degrees3/1 -> Mux10/2
  Demux1/1 -> Mux9/2
  x_ist/1 -> Demux1/1
  Demux/3 -> Radians to Degrees/1

== system PKM_Planar_Testbench_2018/Visualization/Subsystem3 ==
  x_soll : Inport
  x_ist : Inport  Port=2
  Demux : Demux  Outputs=3
  Demux1 : Demux  Outputs=3
  Mux10 : Mux  Inputs=2
  Mux9 : Mux
  Radians to Degrees : simulink_extras/Transformations/Radians to Degrees
  Radians to Degrees3 : simulink_extras/Transformations/Radians to Degrees
  pos_soll_ist : Outport
  ori_soll_ist_deg : Outport  Port=2
  wires:
  Demux/3 -> Radians to Degrees/1
  x_ist/1 -> Demux1/1
  Demux1/1 -> Mux9/2
  Radians to Degrees3/1 -> Mux10/2
  Demux1/2 -> Mux9/4
  Demux1/3 -> Radians to Degrees3/1
  Demux/1 -> Mux9/1
  Demux/2 -> Mux9/3
  Radians to Degrees/1 -> Mux10/1
  x_soll/1 -> Demux/1
  Mux10/1 -> ori_soll_ist_deg/1
  Mux9/1 -> pos_soll_ist/1

== system PKM_Planar_Testbench_2018/Visualization/Subsystem4 ==
  In1 : Inport
  In2 : Inport  Port=2
  Demux : Demux  Outputs=3
  Mux9 : Mux  Inputs=2
  Radians to Degrees : simulink_extras/Transformations/Radians to Degrees
  Sum : Sum  Inputs=|+-
  Out1 : Outport
  Degrees out : Outport  Port=2
  wires:
  In2/1 -> Sum/2
  Sum/1 -> Demux/1
  Demux/1 -> Mux9/1
  Mux9/1 -> Out1/1
  Demux/2 -> Mux9/2
  Demux/3 -> Radians to Degrees/1
  In1/1 -> Sum/1
  Radians to Degrees/1 -> Degrees out/1

== system PKM_Planar_Testbench_2018/Visualization/Subsystem5 ==
  In1 : Inport
  In2 : Inport  Port=2
  Demux : Demux  Outputs=3
  Mux9 : Mux  Inputs=2
  Radians to Degrees : simulink_extras/Transformations/Radians to Degrees
  Sum : Sum  Inputs=|+-
  Out1 : Outport
  Degrees out : Outport  Port=2
  wires:
  Radians to Degrees/1 -> Degrees out/1
  In1/1 -> Sum/1
  Demux/3 -> Radians to Degrees/1
  Demux/2 -> Mux9/2
  Mux9/1 -> Out1/1
  Demux/1 -> Mux9/1
  Sum/1 -> Demux/1
  In2/1 -> Sum/2

== system PKM_Planar_Testbench_2018/Visualization/Subsystem6 ==
  In1 : Inport
  In2 : Inport  Port=2
  Demux : Demux  Outputs=3
  Mux9 : Mux  Inputs=2
  Radians to Degrees : simulink_extras/Transformations/Radians to Degrees
  Sum : Sum  Inputs=|+-
  Out1 : Outport
  Degrees out : Outport  Port=2
  wires:
  In2/1 -> Sum/2
  Sum/1 -> Demux/1
  Demux/1 -> Mux9/1
  Mux9/1 -> Out1/1
  Demux/2 -> Mux9/2
  Demux/3 -> Radians to Degrees/1
  In1/1 -> Sum/1
  Radians to Degrees/1 -> Degrees out/1

== system PKM_Planar_Testbench_2018/Visualization/TP1_impl ==
  u_raw : Inport
  Constant16 : Constant  Value=param.fz_lp  SampleTime=-1
  Delay5 : Delay  DelayLength=1  InitialCondition=zeros(3,1)
  Delay6 : Delay  DelayLength=1  InitialCondition=zeros(3,1)
  MATLAB Function16 : MATLAB Function  TreatAsAtomicUnit=on
  "TP1_scope " : Scope  NumInputPorts=5
  u_filt : Outport
  not_defined_nan : Outport  Port=2
  wires:
  Delay5/1 -> "TP1_scope "/2, MATLAB Function16/2(u_prev)
  u_raw/1 -> Delay5/1, "TP1_scope "/1, MATLAB Function16/1(u_raw)
  MATLAB Function16/1(u_filt) -> "TP1_scope "/4, u_filt/1, Delay6/1
  Constant16/1 -> "TP1_scope "/3, MATLAB Function16/3(a)
  Delay6/1 -> "TP1_scope "/5, MATLAB Function16/4(y_prev)
  MATLAB Function16/2(not_defined_nan) -> not_defined_nan/1

== system PKM_Planar_Testbench_2018/Communication/Klemmen zu Simulink/Uint in double ==
  pos_raw : Inport
  current_raw : Inport  Port=2
  Delay1 : Delay  DelayLength=1
  Delay4 : Delay  DelayLength=1
  MATLAB Function1 : MATLAB Function  TreatAsAtomicUnit=on
  MATLAB Function2 : MATLAB Function  TreatAsAtomicUnit=on
  Position_i1 : Gain  Gain=(2*pi)/(2^(20))  ParamDataTypeStr=float('double')  OutDataTypeStr=float('double')
  Sum1 : Sum  Inputs=|+-
  Torque_i1 : Gain  Gain=(11.3*16.5)/3280  ParamDataTypeStr=float('double')  OutDataTypeStr=float('double')
  offset_s1 : Constant  Value=4.2950e+09  SampleTime=0.001
  pos_Achse12 : DataTypeConversion  OutDataTypeStr=double  SaturateOnIntegerOverflow=off  RndMeth=Floor
  pos : Outport
  vel : Outport  Port=2
  acc : Outport  Port=3
  tau : Outport  Port=4
  wires:
  Position_i1/1 -> Delay1/1, MATLAB Function1/1(u), pos/1
  MATLAB Function2/1(y) -> Torque_i1/1
  [t_sample] -> MATLAB Function1/4(t_sample)
  Delay4/1 -> MATLAB Function1/3(prev_vel)
  pos_raw/1 -> pos_Achse12/1
  MATLAB Function1/1(vel) -> Delay4/1, vel/1  "dq"
  Delay1/1 -> MATLAB Function1/2(prev_pos)
  current_raw/1 -> MATLAB Function2/1(u_uint)
  MATLAB Function1/2(acc) -> acc/1
  Torque_i1/1 -> tau/1  "tau_mess_RD1"
  offset_s1/1 -> Sum1/2
  pos_Achse12/1 -> Sum1/1
  Sum1/1 -> Position_i1/1

== system PKM_Planar_Testbench_2018/Communication/Klemmen zu Simulink/int in double ==
  pos_raw : Inport
  current_raw : Inport  Port=2
  Constant : Constant  Value=param.t_sample  SampleTime=-1
  Delay1 : Delay  DelayLength=1  InitialCondition=param.offset_qa1_rad
  Delay4 : Delay  DelayLength=1
  MATLAB Function1 : MATLAB Function  TreatAsAtomicUnit=on
  Position_i1 : Gain  Gain=(2*pi)/(2^(20))  ParamDataTypeStr=float('double')  OutDataTypeStr=float('double')
  Sum1 : Sum  Inputs=|+-
  Torque_i1 : Gain  Gain=(6.021*16.5)/3280  ParamDataTypeStr=float('double')  OutDataTypeStr=float('double')
  int16_2_double : DataTypeConversion  OutDataTypeStr=double  SaturateOnIntegerOverflow=off  RndMeth=Floor
  offset_s1 : Constant  Value=param.offset_qa1_rad  SampleTime=-1
  pos_Achse12 : DataTypeConversion  OutDataTypeStr=double  SaturateOnIntegerOverflow=off  RndMeth=Floor
  pos : Outport
  vel : Outport  Port=2
  acc : Outport  Port=3
  tau : Outport  Port=4
  wires:
  current_raw/1 -> int16_2_double/1
  Constant/1 -> MATLAB Function1/4(t_sample)
  Delay4/1 -> MATLAB Function1/3(prev_vel)
  pos_raw/1 -> pos_Achse12/1
  MATLAB Function1/1(vel) -> Delay4/1, vel/1  "dq"
  Delay1/1 -> MATLAB Function1/2(prev_pos)
  MATLAB Function1/2(acc) -> acc/1
  Torque_i1/1 -> tau/1  "tau_mess_RD1"
  pos_Achse12/1 -> Position_i1/1
  offset_s1/1 -> Sum1/2
  Position_i1/1 -> Sum1/1
  Sum1/1 -> pos/1, Delay1/1, MATLAB Function1/1(u)
  int16_2_double/1 -> Torque_i1/1
